simulink model "control"  (R2016b)
settings: Solver=VariableStepAuto  StartTime=0.0  StopTime=10.0  RelTol=1e-3
libraries: legoev3lib x4
settings Model: Creator=Nexel  LastModifiedBy=Nexel

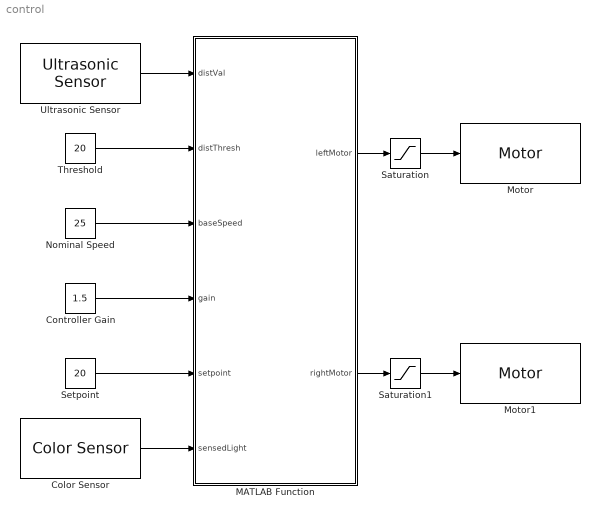
== system control ==
  Color Sensor : legoev3lib/Color Sensor  portNumber=1  mode=Color  sampleTime=0.1
  "Controller Gain " : Constant  Value=1.5
  MATLAB Function : MATLAB Function  TreatAsAtomicUnit=on
  Motor : legoev3lib/Motor  sportNumber=A  sstopAction=Brake
  Motor1 : legoev3lib/Motor  sportNumber=A  sstopAction=Brake
  "Nominal Speed " : Constant  Value=25
  Saturation : Saturate  UpperLimit=100  LowerLimit=-100
  Saturation1 : Saturate  UpperLimit=100  LowerLimit=-100
  Setpoint : Constant  Value=20
  "Threshold " : Constant  Value=20
  Ultrasonic Sensor : legoev3lib/Ultrasonic Sensor  PortNumber=1  sampleTime=0.1
  wires:
  Saturation/1 -> Motor/1
  Saturation1/1 -> Motor1/1
  Ultrasonic Sensor/1 -> MATLAB Function/1(distVal)
  "Threshold "/1 -> MATLAB Function/2(distThresh)
  "Nominal Speed "/1 -> MATLAB Function/3(baseSpeed)
  "Controller Gain "/1 -> MATLAB Function/4(gain)
  Setpoint/1 -> MATLAB Function/5(setpoint)
  Color Sensor/1 -> MATLAB Function/6(sensedLight)
  MATLAB Function/1(leftMotor) -> Saturation/1
  MATLAB Function/2(rightMotor) -> Saturation1/1

== matlab function control/MATLAB Function ==
  data: distVal input; leftMotor output; distThresh input; baseSpeed input; gain input; setpoint input; sensedLight input; rightMotor output
function [leftMotor, rightMotor] = control(distVal, distThresh, baseSpeed, gain, setpoint, sensedLight)
    %#codegen
    if distVal > distThresh % Compare obstruction distance to threshold
         err = sensedLight - setpoint; % Line following logic
         leftMotor = baseSpeed - gain*err;
         rightMotor = baseSpeed + gain*err;
    else
         leftMotor = uint8(0); % Collision avoidance logic
         rightMotor = uint8(0);
end
